simulink subsystem "LoadTypeHandler"  (R2024b)
settings: Solver=VariableStepAuto  StartTime=0.0  StopTime=10.0  RelTol=1e-3
libraries: hdlsllib x6
settings Model: Creator=stefano  LastModifiedBy=stefano

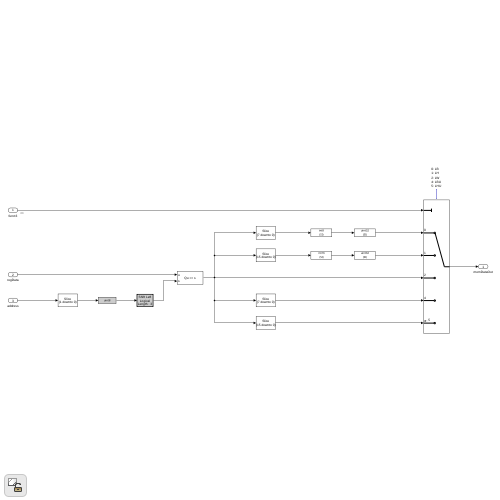
[thumbnail: Simulink's stored preview of the top-level diagram]
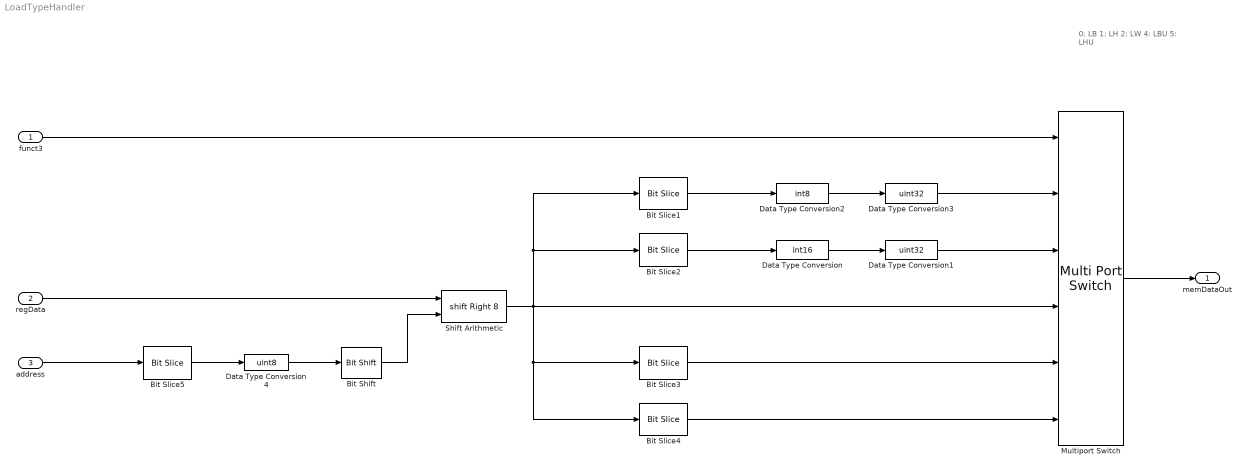
== system LoadTypeHandler ==
  note: 0: LB
      | 1: LH
      | 2: LW
      | 4: LBU
      | 5: LHU
  funct3 : Inport
  regData : Inport  Port=2
  address : Inport  Port=3
  Bit Shift : hdlsllib/Logic and Bit Operations/Bit Shift  mode=Shift Left Logical  N=3
  Bit Slice1 : hdlsllib/Logic and Bit Operations/Bit Slice  lidx=7  ridx=0
  Bit Slice2 : hdlsllib/Logic and Bit Operations/Bit Slice  lidx=15  ridx=0
  Bit Slice3 : hdlsllib/Logic and Bit Operations/Bit Slice  lidx=7  ridx=0
  Bit Slice4 : hdlsllib/Logic and Bit Operations/Bit Slice  lidx=15  ridx=0
  Bit Slice5 : hdlsllib/Logic and Bit Operations/Bit Slice  lidx=1  ridx=0
  Data Type Conversion : DataTypeConversion  OutDataTypeStr=int16  ConvertRealWorld=Stored Integer (SI)  SaturateOnIntegerOverflow=off  RndMeth=Floor
  Data Type Conversion1 : DataTypeConversion  OutDataTypeStr=uint32  ConvertRealWorld=Stored Integer (SI)  SaturateOnIntegerOverflow=off  RndMeth=Floor
  Data Type Conversion2 : DataTypeConversion  OutDataTypeStr=int8  ConvertRealWorld=Stored Integer (SI)  SaturateOnIntegerOverflow=off  RndMeth=Floor
  Data Type Conversion3 : DataTypeConversion  OutDataTypeStr=uint32  ConvertRealWorld=Stored Integer (SI)  SaturateOnIntegerOverflow=off  RndMeth=Floor
  Data Type Conversion4 : DataTypeConversion  OutDataTypeStr=uint8  SaturateOnIntegerOverflow=off  RndMeth=Floor
  Multiport Switch : MultiPortSwitch  DataPortOrder=Specify indices  Inputs=5  DataPortIndices={0,1,2,4,5}  DiagnosticForDefault=None  SaturateOnIntegerOverflow=off  InputSameDT=off
  Shift Arithmetic : ArithShift  BitShiftNumberSource=Input port  BitShiftNumber=8  BitShiftDirection=Right
      settings: InputPortMap=u0,p1
  memDataOut : Outport
  wires:
  address/1 -> Bit Slice5/1
  funct3/1 -> Multiport Switch/1
  Bit Slice3/1 -> Multiport Switch/5
  Data Type Conversion4/1 -> Bit Shift/1
  Bit Shift/1 -> Shift Arithmetic/2
  Bit Slice5/1 -> Data Type Conversion4/1
  regData/1 -> Shift Arithmetic/1
  Data Type Conversion2/1 -> Data Type Conversion3/1
  Data Type Conversion3/1 -> Multiport Switch/2
  Data Type Conversion1/1 -> Multiport Switch/3
  Data Type Conversion/1 -> Data Type Conversion1/1
  Bit Slice4/1 -> Multiport Switch/6
  Bit Slice1/1 -> Data Type Conversion2/1
  Shift Arithmetic/1 -> Bit Slice4/1, Bit Slice3/1, Bit Slice2/1, Bit Slice1/1, Multiport Switch/4
  Bit Slice2/1 -> Data Type Conversion/1
  Multiport Switch/1 -> memDataOut/1
